simulink model "pitch_loop"  (R2016b)
settings: Solver=VariableStepAuto  StartTime=0.0  StopTime=10.0  RelTol=1e-3
undefined symbols (not defined in the file): a_theta1, a_theta2, a_theta3, k_d_theta, k_p_theta
settings Model: Creator=geun2  LastModifiedBy=geun2

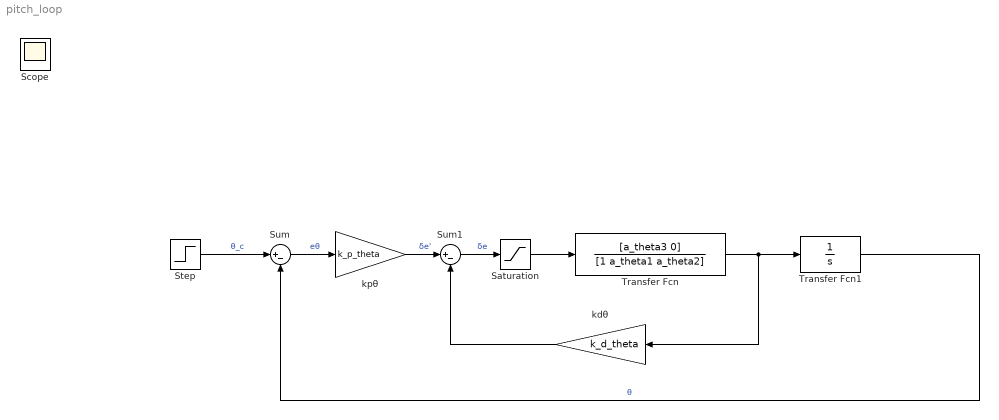
== system pitch_loop ==
  Saturation : Saturate  UpperLimit=45*pi/180  LowerLimit=-45*pi/180
  Step : Step  After=10*pi/180  SampleTime=0
  Sum : Sum  Inputs=|+-
  Sum1 : Sum  Inputs=|+-
  Transfer Fcn : TransferFcn  Numerator=[a_theta3 0]  Denominator=[1 a_theta1 a_theta2]
  Transfer Fcn1 : TransferFcn  Denominator=[1 0]
  kdθ : Gain  Gain=k_d_theta
  kpθ : Gain  Gain=k_p_theta
  Scope : Scope
  wires:
  Sum/1 -> kpθ/1  "eθ"
  kpθ/1 -> Sum1/1  "δe'"
  Sum1/1 -> Saturation/1  "δe"
  Transfer Fcn/1 -> Transfer Fcn1/1, kdθ/1
  Transfer Fcn1/1 -> Sum/2  "θ"
  kdθ/1 -> Sum1/2
  Step/1 -> Sum/1  "θ_c"
  Saturation/1 -> Transfer Fcn/1
